simulink model "CL"  (R2025b)
settings: Solver=VariableStepAuto  StartTime=0.0  StopTime=10.0  RelTol=1e-3
values from neighbouring files (symbols this model uses):
  plant = ss(a,b,c,d)    [data_avion_lat.m]
undefined symbols (not defined in the file or in its folder): H, K
settings Model: Creator=flo  LastModifiedBy=flo

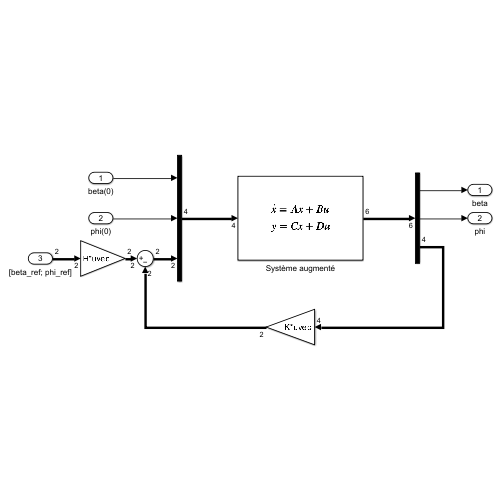
[thumbnail: Simulink's stored preview of the top-level diagram]
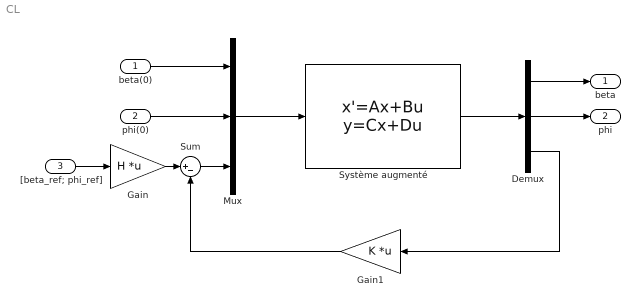
== system CL ==
  beta(0) : Inport
  phi(0) : Inport  Port=2
  "[beta_ref; phi_ref]" : Inport  Port=3
  Demux : Demux  Outputs=[1;1;4]
  Gain : Gain  Gain=H  Multiplication=Matrix(K*u) (u vector)
  Gain1 : Gain  Gain=K  Multiplication=Matrix(K*u) (u vector)
  Mux : Mux  Inputs=[1;1;2]
  Sum : Sum  Inputs=|+-
  Système augmenté : StateSpace  A=plant.a  B=[[1 0; 0 0; 0 0; 0 1] plant.b]  C=[[1 0 0 0; 0 0 0 1]; plant.c]  D=[zeros(2,4); zeros(4,2) plant.d]  InitialCondition=0
  beta : Outport
  phi : Outport  Port=2
  wires:
  Mux/1 -> Système augmenté/1
  beta(0)/1 -> Mux/1
  phi(0)/1 -> Mux/2
  "[beta_ref; phi_ref]"/1 -> Gain/1
  Système augmenté/1 -> Demux/1
  Demux/2 -> phi/1
  Demux/1 -> beta/1
  Demux/3 -> Gain1/1
  Gain/1 -> Sum/1
  Sum/1 -> Mux/3
  Gain1/1 -> Sum/2
